simulink model "Modello_Irb1300"  (R2024a)
settings: Solver=VariableStepAuto  StartTime=0.0  StopTime=37  RelTol=1e-3
undefined symbols (not defined in the file or in its folder): DiscIntNeverNeededParam
libraries: vrlib x3, simulink x1
(part 1 of 2)
settings Model: Creator=giaki  LastModifiedBy=giaki

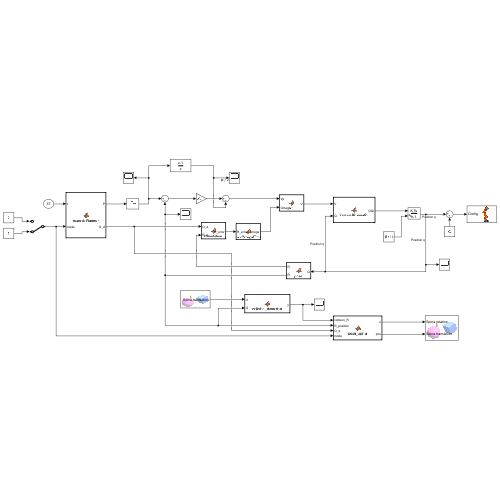
[thumbnail: Simulink's stored preview of the top-level diagram]
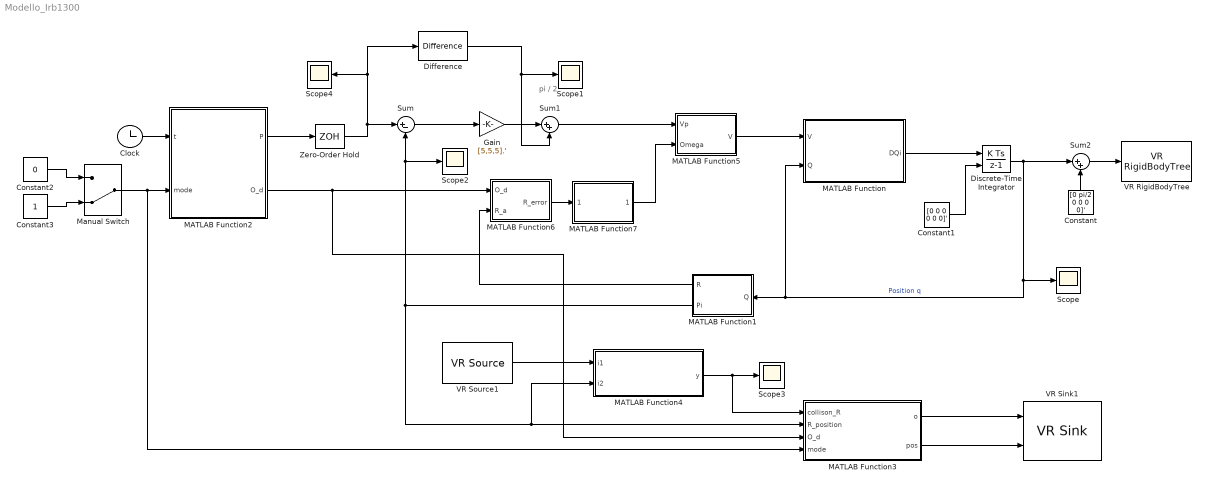
== system Modello_Irb1300 ==
  note: pi / 2
  Clock : Clock
  Constant : Constant  Value=[0 pi/2 0 0 0 0]'
  Constant1 : Constant  Value=[0 0 0 0 0 0]'
  Constant2 : Constant  Value=0
  Constant3 : Constant
  Difference : simulink/Discrete/Difference  ICPrevInput=[0.66, 0, 1.015].'  OutMin=[]  OutMax=[]  OutDataType=fixdt(1, 16)  OutScaling=2^-10  DoSatur=off
  Discrete-Time Integrator : DiscreteIntegrator  InitialConditionSource=external  SampleTime=-1  OutMin=[2]  ICPrevOutput=DiscIntNeverNeededParam  ICPrevScaledInput=DiscIntNeverNeededParam
  Gain : Gain  Gain=[5,5,5].'
  MATLAB Function : MATLAB Function  TreatAsAtomicUnit=on
  MATLAB Function1 : MATLAB Function  TreatAsAtomicUnit=on
  MATLAB Function2 : MATLAB Function  TreatAsAtomicUnit=on
  MATLAB Function3 : MATLAB Function  TreatAsAtomicUnit=on
  MATLAB Function4 : MATLAB Function  TreatAsAtomicUnit=on
  MATLAB Function5 : MATLAB Function  TreatAsAtomicUnit=on
  MATLAB Function6 : MATLAB Function  TreatAsAtomicUnit=on
  MATLAB Function7 : MATLAB Function  TreatAsAtomicUnit=on
  Manual Switch : ManualSwitch  CurrentSetting=0
  Scope{,1..4} (5 alike) : Scope
  Sum : Sum  Inputs=|+-
  Sum1 : Sum  Inputs=|++
  Sum2 : Sum  Inputs=|++
  VR RigidBodyTree : vrlib/VR RigidBodyTree  VrmlFile=robot_scene_2.x3d  RBT=Irb1300  useRBT=on  Ts=0.1  ForceViewerOpen=on
  VR Sink1 : vrlib/VR Sink  InstantiateOnLoad=on  SampleTime=0.1  ViewEnable=on  RemoteChange=off  RemoteView=off  FieldsWritten=Spina.rotation.4.1.1.double#Spina.translation.3.1.1.double  WorldFileName=robot_scene_2.x3d  WorldDescription=Simple Robot Scene  AutoView=off  VideoDimensions=[]  AllowVariableSize=off
  VR Source1 : vrlib/VR Source  InstantiateOnLoad=on  SampleTime=0.1  ViewEnable=on  RemoteChange=off  RemoteView=off  FieldsRead=Spina.translation.1.3.1.double  WorldFileName=robot_scene_2.x3d  WorldDescription=Simple Robot Scene  AutoView=off  VideoDimensions=[]  AllowVariableSize=off
  Zero-Order Hold : ZeroOrderHold  SampleTime=0.05
  wires:
  Discrete-Time Integrator/1 -> Sum2/1, Scope/1, MATLAB Function/2(Q), MATLAB Function1/1(Q)  "Position q"
  Constant/1 -> Sum2/2
  Constant1/1 -> Discrete-Time Integrator/2
  Sum2/1 -> VR RigidBodyTree/1
  Difference/1 -> Sum1/2, Scope1/1
  Clock/1 -> MATLAB Function2/1(t)
  MATLAB Function/1(DQi) -> Discrete-Time Integrator/1
  Gain/1 -> Sum1/1
  MATLAB Function4/1(y) -> MATLAB Function3/1(collison_R), Scope3/1
  VR Source1/1 -> MATLAB Function4/1(i1)
  MATLAB Function2/1(P) -> Zero-Order Hold/1
  MATLAB Function3/2(pos) -> VR Sink1/2
  Zero-Order Hold/1 -> Scope4/1, Difference/1, Sum/1
  Sum/1 -> Gain/1
  MATLAB Function1/1(R) -> MATLAB Function6/2(R_a)
  Sum1/1 -> MATLAB Function5/1(Vp)
  MATLAB Function5/1(V) -> MATLAB Function/1(V)
  MATLAB Function6/1(R_error) -> MATLAB Function7/1(R_error)
  MATLAB Function7/1(omega) -> MATLAB Function5/2(Omega)
  MATLAB Function1/2(Pi) -> Sum/2, Scope2/1, MATLAB Function4/2(i2), MATLAB Function3/2(R_position)
  MATLAB Function2/2(O_d) -> MATLAB Function3/3(O_d), MATLAB Function6/1(O_d)
  MATLAB Function3/1(o) -> VR Sink1/1
  Manual Switch/1 -> MATLAB Function3/4(mode), MATLAB Function2/2(mode)
  Constant2/1 -> Manual Switch/1
  Constant3/1 -> Manual Switch/2

== matlab function Modello_Irb1300/MATLAB Function1 ==
  data: R output; Q input; Pi output


function [R,Pi] = posa(Q)

th1 = Q(1);
th2 = Q(2);
th3 = Q(3);
th4 = Q(4);
th5 = Q(5);
th6 = Q(6);

% Matrice di trasformazione 4x4 calcolata nella posizione Q
T = [
    [sin(th6)*(cos(th4)*sin(th1) + sin(th4)*(cos(th1)*sin(th3)*sin(th2 + pi/2) - cos(th1)*cos(th3)*cos(th2 + pi/2))) + cos(th6)*(cos(th5)*(sin(th1)*sin(th4) - cos(th4)*(cos(th1)*sin(th3)*sin(th2 + pi/2) - cos(th1)*cos(th3)*cos(th2 + pi/2))) - sin(th5)*(cos(th1)*cos(th3)*sin(th2 + pi/2) + cos(th1)*cos(th2 + pi/2)*sin(th3))), cos(th6)*(cos(th4)*sin(th1) + sin(th4)*(cos(th1)*sin(th3)*sin(th2 + pi/2) - cos(th1)*cos(th3)*cos(th2 + pi/2))) - sin(th6)*(cos(th5)*(sin(th1)*sin(th4) - cos(th4)*(cos(th1)*sin(th3)*sin(th2 + pi/2) - cos(th1)*cos(th3)*cos(th2 + pi/2))) - sin(th5)*(cos(th1)*cos(th3)*sin(th2 + pi/2) + cos(th1)*cos(th2 + pi/2)*sin(th3))), sin(th5)*(sin(th1)*sin(th4) - cos(th4)*(cos(th1)*sin(th3)*sin(th2 + pi/2) - cos(th1)*cos(th3)*cos(th2 + pi/2))) + cos(th5)*(cos(th1)*cos(th3)*sin(th2 + pi/2) + cos(th1)*cos(th2 + pi/2)*sin(th3)), cos(th1)/20 + (17*cos(th1)*cos(th2 + pi/2))/40 + (9*sin(th5)*(sin(th1)*sin(th4) - cos(th4)*(cos(th1)*sin(th3)*sin(th2 + pi/2) - cos(th1)*cos(th3)*cos(th2 + pi/2))))/50 + (9*cos(th5)*(cos(th1)*cos(th3)*sin(th2 + pi/2) + cos(th1)*cos(th2 + pi/2)*sin(th3)))/50 + (17*cos(th1)*cos(th3)*sin(th2 + pi/2))/40 + (17*cos(th1)*cos(th2 + pi/2)*sin(th3))/40 - (cos(th1)*sin(th3)*sin(th2 + pi/2))/25 + (cos(th1)*cos(th3)*cos(th2 + pi/2))/25]
    [-sin(th6)*(cos(th1)*cos(th4) + sin(th4)*(cos(th3)*cos(th2 + pi/2)*sin(th1) - sin(th1)*sin(th3)*sin(th2 + pi/2))) - cos(th6)*(cos(th5)*(cos(th1)*sin(th4) - cos(th4)*(cos(th3)*cos(th2 + pi/2)*sin(th1) - sin(th1)*sin(th3)*sin(th2 + pi/2))) + sin(th5)*(cos(th3)*sin(th1)*sin(th2 + pi/2) + cos(th2 + pi/2)*sin(th1)*sin(th3))), sin(th6)*(cos(th5)*(cos(th1)*sin(th4) - cos(th4)*(cos(th3)*cos(th2 + pi/2)*sin(th1) - sin(th1)*sin(th3)*sin(th2 + pi/2))) + sin(th5)*(cos(th3)*sin(th1)*sin(th2 + pi/2) + cos(th2 + pi/2)*sin(th1)*sin(th3))) - cos(th6)*(cos(th1)*cos(th4) + sin(th4)*(cos(th3)*cos(th2 + pi/2)*sin(th1) - sin(th1)*sin(th3)*sin(th2 + pi/2))), cos(th5)*(cos(th3)*sin(th1)*sin(th2 + pi/2) + cos(th2 + pi/2)*sin(th1)*sin(th3)) - sin(th5)*(cos(th1)*sin(th4) - cos(th4)*(cos(th3)*cos(th2 + pi/2)*sin(th1) - sin(th1)*sin(th3)*sin(th2 + pi/2))), sin(th1)/20 + (17*cos(th2 + pi/2)*sin(th1))/40 - (9*sin(th5)*(cos(th1)*sin(th4) - cos(th4)*(cos(th3)*cos(th2 + pi/2)*sin(th1) - sin(th1)*sin(th3)*sin(th2 + pi/2))))/50 + (9*cos(th5)*(cos(th3)*sin(th1)*sin(th2 + pi/2) + cos(th2 + pi/2)*sin(th1)*sin(th3)))/50 + (cos(th3)*cos(th2 + pi/2)*sin(th1))/25 + (17*cos(th3)*sin(th1)*sin(th2 + pi/2))/40 + (17*cos(th2 + pi/2)*sin(th1)*sin(th3))/40 - (sin(th1)*sin(th3)*sin(th2 + pi/2))/25]
    [cos(th6)*(sin(th5)*(cos(th3)*cos(th2 + pi/2) - sin(th3)*sin(th2 + pi/2)) + cos(th4)*cos(th5)*(cos(th3)*sin(th2 + pi/2) + cos(th2 + pi/2)*sin(th3))) - sin(th4)*sin(th6)*(cos(th3)*sin(th2 + pi/2) + cos(th2 + pi/2)*sin(th3)), -sin(th6)*(sin(th5)*(cos(th3)*cos(th2 + pi/2) - sin(th3)*sin(th2 + pi/2)) + cos(th4)*cos(th5)*(cos(th3)*sin(th2 + pi/2) + cos(th2 + pi/2)*sin(th3))) - cos(th6)*sin(th4)*(cos(th3)*sin(th2 + pi/2) + cos(th2 + pi/2)*sin(th3)), cos(th4)*sin(th5)*(cos(th3)*sin(th2 + pi/2) + cos(th2 + pi/2)*sin(th3)) - cos(th5)*(cos(th3)*cos(th2 + pi/2) - sin(th3)*sin(th2 + pi/2)), (17*sin(th2 + pi/2))/40 - (17*cos(th3)*cos(th2 + pi/2))/40 + (cos(th3)*sin(th2 + pi/2))/25 + (cos(th2 + pi/2)*sin(th3))/25 + (17*sin(th3)*sin(th2 + pi/2))/40 - (9*cos(th5)*(cos(th3)*cos(th2 + pi/2) - sin(th3)*sin(th2 + pi/2)))/50 + (9*cos(th4)*sin(th5)*(cos(th3)*sin(th2 + pi/2) + cos(th2 + pi/2)*sin(th3)))/50 + 68/125]
    [0, 0, 0, 1]
];

% Estrai la posizione (3x1)
Pi_position = T(1:3, 4);

% Estrai la matrice di rotazione (3x3)
R = T(1:3, 1:3);

% % Calcola Roll, Pitch, Yaw dalla matrice di rotazione
% roll = atan2(R(3,2), R(3,3));   % Roll (x)
% pitch = atan2(-R(3,1), sqrt(R(3,2)^2 + R(3,3)^2));  % Pitch (y)
% yaw = atan2(R(2,1), R(1,1));    % Yaw (z)
% 
% % Mantieni roll, pitch, yaw nel range [-π, π]
% roll = wrapToPi(roll);
% pitch = wrapToPi(pitch);
% yaw = wrapToPi(yaw);

% Restituisci la posizione e l'orientamento come un vettore 6x1
%Pi = [Pi_position; roll; pitch; yaw];
%Pi = [Pi_position; R(:,3)];
Pi = [Pi_position];
% end













% function Pi = posa(Q)
% 
% th1 = Q(1);
% th2 = Q(2);
% th3 = Q(3);
% th4 = Q(4);
% th5 = Q(5);
% th6 = Q(6);
% 
% % matrix 4x4 evaluated in the position Q
% % matriceUtilizzata T06 calcolata con la terna di riferimento posizionata
% % sul punto di aggancio della pinza 
% T = [
% [  sin(th6)*(cos(th4)*sin(th1) + sin(th4)*(cos(th1)*sin(th3)*sin(th2 + pi/2) - cos(th1)*cos(th3)*cos(th2 + pi/2))) + cos(th6)*(cos(th5)*(sin(th1)*sin(th4) - cos(th4)*(cos(th1)*sin(th3)*sin(th2 + pi/2) - cos(th1)*cos(th3)*cos(th2 + pi/2))) - sin(th5)*(cos(th1)*cos(th3)*sin(th2 + pi/2) + cos(th1)*cos(th2 + pi/2)*sin(th3))), cos(th6)*(cos(th4)*sin(th1) + sin(th4)*(cos(th1)*sin(th3)*sin(th2 + pi/2) - cos(th1)*cos(th3)*cos(th2 + pi/2))) - sin(th6)*(cos(th5)*(sin(th1)*sin(th4) - cos(th4)*(cos(th1)*sin(th3)*sin(th2 + pi/2) - cos(th1)*cos(th3)*cos(th2 + pi/2))) - sin(th5)*(cos(th1)*cos(th3)*sin(th2 + pi/2) + cos(th1)*cos(th2 + pi/2)*sin(th3))), sin(th5)*(sin(th1)*sin(th4) - cos(th4)*(cos(th1)*sin(th3)*sin(th2 + pi/2) - cos(th1)*cos(th3)*cos(th2 + pi/2))) + cos(th5)*(cos(th1)*cos(th3)*sin(th2 + pi/2) + cos(th1)*cos(th2 + pi/2)*sin(th3)), cos(th1)/20 + (17*cos(th1)*cos(th2 + pi/2))/40 + (9*sin(th5)*(sin(th1)*sin(th4) - cos(th4)*(cos(th1)*sin(th3)*sin(th2 + pi/2) - cos(th1)*cos(th3)*cos(th2 + pi/2))))/50 + (9*cos(th5)*(cos(th1)*cos(th3)*sin(th2 + pi/2) + cos(th1)*cos(th2 + pi/2)*sin(th3)))/50 + (17*cos(th1)*cos(th3)*sin(th2 + pi/2))/40 + (17*cos(th1)*cos(th2 + pi/2)*sin(th3))/40 - (cos(th1)*sin(th3)*sin(th2 + pi/2))/25 + (cos(th1)*cos(th3)*cos(th2 + pi/2))/25]
% [- sin(th6)*(cos(th1)*cos(th4) + sin(th4)*(cos(th3)*cos(th2 + pi/2)*sin(th1) - sin(th1)*sin(th3)*sin(th2 + pi/2))) - cos(th6)*(cos(th5)*(cos(th1)*sin(th4) - cos(th4)*(cos(th3)*cos(th2 + pi/2)*sin(th1) - sin(th1)*sin(th3)*sin(th2 + pi/2))) + sin(th5)*(cos(th3)*sin(th1)*sin(th2 + pi/2) + cos(th2 + pi/2)*sin(th1)*sin(th3))), sin(th6)*(cos(th5)*(cos(th1)*sin(th4) - cos(th4)*(cos(th3)*cos(th2 + pi/2)*sin(th1) - sin(th1)*sin(th3)*sin(th2 + pi/2))) + sin(th5)*(cos(th3)*sin(th1)*sin(th2 + pi/2) + cos(th2 + pi/2)*sin(th1)*sin(th3))) - cos(th6)*(cos(th1)*cos(th4) + sin(th4)*(cos(th3)*cos(th2 + pi/2)*sin(th1) - sin(th1)*sin(th3)*sin(th2 + pi/2))), cos(th5)*(cos(th3)*sin(th1)*sin(th2 + pi/2) + cos(th2 + pi/2)*sin(th1)*sin(th3)) - sin(th5)*(cos(th1)*sin(th4) - cos(th4)*(cos(th3)*cos(th2 + pi/2)*sin(th1) - sin(th1)*sin(th3)*sin(th2 + pi/2))), sin(th1)/20 + (17*cos(th2 + pi/2)*sin(th1))/40 - (9*sin(th5)*(cos(th1)*sin(th4) - cos(th4)*(cos(th3)*cos(th2 + pi/2)*sin(th1) - sin(th1)*sin(th3)*sin(th2 + pi/2))))/50 + (9*cos(th5)*(cos(th3)*sin(th1)*sin(th2 + pi/2) + cos(th2 + pi/2)*sin(th1)*sin(th3)))/50 + (cos(th3)*cos(th2 + pi/2)*sin(th1))/25 + (17*cos(th3)*sin(th1)*sin(th2 + pi/2))/40 + (17*cos(th2 + pi/2)*sin(th1)*sin(th3))/40 - (sin(th1)*sin(th3)*sin(th2 + pi/2))/25]
% [                                                                                                    cos(th6)*(sin(th5)*(cos(th3)*cos(th2 + pi/2) - sin(th3)*sin(th2 + pi/2)) + cos(th4)*cos(th5)*(cos(th3)*sin(th2 + pi/2) + cos(th2 + pi/2)*sin(th3))) - sin(th4)*sin(th6)*(cos(th3)*sin(th2 + pi/2) + cos(th2 + pi/2)*sin(th3)),                                                                                                 - sin(th6)*(sin(th5)*(cos(th3)*cos(th2 + pi/2) - sin(th3)*sin(th2 + pi/2)) + cos(th4)*cos(th5)*(cos(th3)*sin(th2 + pi/2) + cos(th2 + pi/2)*sin(th3))) - cos(th6)*sin(th4)*(cos(th3)*sin(th2 + pi/2) + cos(th2 + pi/2)*sin(th3)),                                                           cos(th4)*sin(th5)*(cos(th3)*sin(th2 + pi/2) + cos(th2 + pi/2)*sin(th3)) - cos(th5)*(cos(th3)*cos(th2 + pi/2) - sin(th3)*sin(th2 + pi/2)),                                                                                                             (17*sin(th2 + pi/2))/40 - (17*cos(th3)*cos(th2 + pi/2))/40 + (cos(th3)*sin(th2 + pi/2))/25 + (cos(th2 + pi/2)*sin(th3))/25 + (17*sin(th3)*sin(th2 + pi/2))/40 - (9*cos(th5)*(cos(th3)*cos(th2 + pi/2) - sin(th3)*sin(th2 + pi/2)))/50 + (9*cos(th4)*sin(th5)*(cos(th3)*sin(th2 + pi/2) + cos(th2 + pi/2)*sin(th3)))/50 + 68/125]
% [                                                                                                                                                                                                                                                                                                                                0,                                                                                                                                                                                                                                                                                                                               0,                                                                                                                                                                                                  0,                                                                                                                                                                                                                                                                                                                                                                                                                                           1]
%  ];
% 
% % T = [
% % [  sin(th6)*(cos(th4)*sin(th1) + sin(th4)*(cos(th1)*sin(th3)*sin(th2 + pi/2) - cos(th1)*cos(th3)*cos(th2 + pi/2))) + cos(th6)*(cos(th5)*(sin(th1)*sin(th4) - cos(th4)*(cos(th1)*sin(th3)*sin(th2 + pi/2) - cos(th1)*cos(th3)*cos(th2 + pi/2))) - sin(th5)*(cos(th1)*cos(th3)*sin(th2 + pi/2) + cos(th1)*cos(th2 + pi/2)*sin(th3))), cos(th6)*(cos(th4)*sin(th1) + sin(th4)*(cos(th1)*sin(th3)*sin(th2 + pi/2) - cos(th1)*cos(th3)*cos(th2 + pi/2))) - sin(th6)*(cos(th5)*(sin(th1)*sin(th4) - cos(th4)*(cos(th1)*sin(th3)*sin(th2 + pi/2) - cos(th1)*cos(th3)*cos(th2 + pi/2))) - sin(th5)*(cos(th1)*cos(th3)*sin(th2 + pi/2) + cos(th1)*cos(th2 + pi/2)*sin(th3))), sin(th5)*(sin(th1)*sin(th4) - cos(th4)*(cos(th1)*sin(th3)*sin(th2 + pi/2) - cos(th1)*cos(th3)*cos(th2 + pi/2))) + cos(th5)*(cos(th1)*cos(th3)*sin(th2 + pi/2) + cos(th1)*cos(th2 + pi/2)*sin(th3)), cos(th1)/20 + (17*cos(th1)*cos(th2 + pi/2))/40 + (9*sin(th5)*(sin(th1)*sin(th4) - cos(th4)*(cos(th1)*sin(th3)*sin(th2 + pi/2) - cos(th1)*cos(th3)*cos(th2 + pi/2))))/100 + (9*cos(th5)*(cos(th1)*cos(th3)*sin(th2 + pi/2) + cos(th1)*cos(th2 + pi/2)*sin(th3)))/100 + (17*cos(th1)*cos(th3)*sin(th2 + pi/2))/40 + (17*cos(th1)*cos(th2 + pi/2)*sin(th3))/40 - (cos(th1)*sin(th3)*sin(th2 + pi/2))/25 + (cos(th1)*cos(th3)*cos(th2 + pi/2))/25]
% % [- sin(th6)*(cos(th1)*cos(th4) + sin(th4)*(cos(th3)*cos(th2 + pi/2)*sin(th1) - sin(th1)*sin(th3)*sin(th2 + pi/2))) - cos(th6)*(cos(th5)*(cos(th1)*sin(th4) - cos(th4)*(cos(th3)*cos(th2 + pi/2)*sin(th1) - sin(th1)*sin(th3)*sin(th2 + pi/2))) + sin(th5)*(cos(th3)*sin(th1)*sin(th2 + pi/2) + cos(th2 + pi/2)*sin(th1)*sin(th3))), sin(th6)*(cos(th5)*(cos(th1)*sin(th4) - cos(th4)*(cos(th3)*cos(th2 + pi/2)*sin(th1) - sin(th1)*sin(th3)*sin(th2 + pi/2))) + sin(th5)*(cos(th3)*sin(th1)*sin(th2 + pi/2) + cos(th2 + pi/2)*sin(th1)*sin(th3))) - cos(th6)*(cos(th1)*cos(th4) + sin(th4)*(cos(th3)*cos(th2 + pi/2)*sin(th1) - sin(th1)*sin(th3)*sin(th2 + pi/2))), cos(th5)*(cos(th3)*sin(th1)*sin(th2 + pi/2) + cos(th2 + pi/2)*sin(th1)*sin(th3)) - sin(th5)*(cos(th1)*sin(th4) - cos(th4)*(cos(th3)*cos(th2 + pi/2)*sin(th1) - sin(th1)*sin(th3)*sin(th2 + pi/2))), sin(th1)/20 + (17*cos(th2 + pi/2)*sin(th1))/40 - (9*sin(th5)*(cos(th1)*sin(th4) - cos(th4)*(cos(th3)*cos(th2 + pi/2)*sin(th1) - sin(th1)*sin(th3)*sin(th2 + pi/2))))/100 + (9*cos(th5)*(cos(th3)*sin(th1)*sin(th2 + pi/2) + cos(th2 + pi/2)*sin(th1)*sin(th3)))/100 + (cos(th3)*cos(th2 + pi/2)*sin(th1))/25 + (17*cos(th3)*sin(th1)*sin(th2 + pi/2))/40 + (17*cos(th2 + pi/2)*sin(th1)*sin(th3))/40 - (sin(th1)*sin(th3)*sin(th2 + pi/2))/25]
% % [                                                                                                    cos(th6)*(sin(th5)*(cos(th3)*cos(th2 + pi/2) - sin(th3)*sin(th2 + pi/2)) + cos(th4)*cos(th5)*(cos(th3)*sin(th2 + pi/2) + cos(th2 + pi/2)*sin(th3))) - sin(th4)*sin(th6)*(cos(th3)*sin(th2 + pi/2) + cos(th2 + pi/2)*sin(th3)),                                                                                                 - sin(th6)*(sin(th5)*(cos(th3)*cos(th2 + pi/2) - sin(th3)*sin(th2 + pi/2)) + cos(th4)*cos(th5)*(cos(th3)*sin(th2 + pi/2) + cos(th2 + pi/2)*sin(th3))) - cos(th6)*sin(th4)*(cos(th3)*sin(th2 + pi/2) + cos(th2 + pi/2)*sin(th3)),                                                           cos(th4)*sin(th5)*(cos(th3)*sin(th2 + pi/2) + cos(th2 + pi/2)*sin(th3)) - cos(th5)*(cos(th3)*cos(th2 + pi/2) - sin(th3)*sin(th2 + pi/2)),                                                                                                             (17*sin(th2 + pi/2))/40 - (17*cos(th3)*cos(th2 + pi/2))/40 + (cos(th3)*sin(th2 + pi/2))/25 + (cos(th2 + pi/2)*sin(th3))/25 + (17*sin(th3)*sin(th2 + pi/2))/40 - (9*cos(th5)*(cos(th3)*cos(th2 + pi/2) - sin(th3)*sin(th2 + pi/2)))/100 + (9*cos(th4)*sin(th5)*(cos(th3)*sin(th2 + pi/2) + cos(th2 + pi/2)*sin(th3)))/100 + 68/125]
% % [                                                                                                                                                                                                                                                                                                                                0,                                                                                                                                                                                                                                                                                                                               0,                                                                                                                                                                                                  0,                                                                                                                                                                                                                                                                                                                                                                                                                                             1]
% % ];
% 
% 
% % Estrai la posizione (3x1)
% Pi_position = T(1:3, 4);
% 
% % Estrai la matrice di rotazione (3x3)
% R = T(1:3, 1:3);
% 
% % % Calcola Roll, Pitch, Yaw dalla matrice di rotazione
% roll = atan2(R(3,2), R(3,3));   % Roll (x)
% pitch = atan2(-R(3,1), sqrt(R(3,2)^2 + R(3,3)^2));  % Pitch (y)
% yaw = atan2(R(2,1), R(1,1));    % Yaw (z)
% 
% % Restituisci la posizione e l'orientamento come un vettore 6x1%
% Pi = [Pi_position; roll; pitch; yaw];  % iniziale 
% %Pi = [Pi_position; yaw; pitch; roll];  % Test
% %Pi = [Pi_position; pitch; yaw; roll];
% %Pi = [Pi_position];
% end

== matlab function Modello_Irb1300/MATLAB Function ==
  data: V input; DQi output; Q input
function DQi = inverseKinematic(V,Q)

th1 = Q(1);
th2 = Q(2);
th3 = Q(3);
th4 = Q(4);
th5 = Q(5);
th6 = Q(6);



% cosiderando sia le traslazioni che le orientazioni viene utilizzato il seguente J che si riferisce al jacobiano completo J = Jp + Jo 
J = [
[(9*sin(th5)*(cos(th1)*sin(th4) - cos(th4)*(cos(th3)*cos(th2 + pi/2)*sin(th1) - sin(th1)*sin(th3)*sin(th2 + pi/2))))/50 - (17*cos(th2 + pi/2)*sin(th1))/40 - sin(th1)/20 - (9*cos(th5)*(cos(th3)*sin(th1)*sin(th2 + pi/2) + cos(th2 + pi/2)*sin(th1)*sin(th3)))/50 - (cos(th3)*cos(th2 + pi/2)*sin(th1))/25 - (17*cos(th3)*sin(th1)*sin(th2 + pi/2))/40 - (17*cos(th2 + pi/2)*sin(th1)*sin(th3))/40 + (sin(th1)*sin(th3)*sin(th2 + pi/2))/25, (17*cos(th1)*cos(th3)*cos(th2 + pi/2))/40 - (9*cos(th5)*(cos(th1)*sin(th3)*sin(th2 + pi/2) - cos(th1)*cos(th3)*cos(th2 + pi/2)))/50 - (cos(th1)*cos(th3)*sin(th2 + pi/2))/25 - (cos(th1)*cos(th2 + pi/2)*sin(th3))/25 - (17*cos(th1)*sin(th3)*sin(th2 + pi/2))/40 - (9*cos(th4)*sin(th5)*(cos(th1)*cos(th3)*sin(th2 + pi/2) + cos(th1)*cos(th2 + pi/2)*sin(th3)))/50 - (17*cos(th1)*sin(th2 + pi/2))/40, (17*cos(th1)*cos(th3)*cos(th2 + pi/2))/40 - (cos(th1)*cos(th3)*sin(th2 + pi/2))/25 - (cos(th1)*cos(th2 + pi/2)*sin(th3))/25 - (17*cos(th1)*sin(th3)*sin(th2 + pi/2))/40 - (9*cos(th4)*sin(th5)*(cos(th1)*cos(th3)*sin(th2 + pi/2) + cos(th1)*cos(th2 + pi/2)*sin(th3)))/50 - (9*cos(th5)*(cos(th1)*sin(th3)*sin(th2 + pi/2) - cos(th1)*cos(th3)*cos(th2 + pi/2)))/50,  (9*sin(th5)*(cos(th4)*sin(th1) + sin(th4)*(cos(th1)*sin(th3)*sin(th2 + pi/2) - cos(th1)*cos(th3)*cos(th2 + pi/2))))/50,   (9*cos(th5)*(sin(th1)*sin(th4) - cos(th4)*(cos(th1)*sin(th3)*sin(th2 + pi/2) - cos(th1)*cos(th3)*cos(th2 + pi/2))))/50 - (9*sin(th5)*(cos(th1)*cos(th3)*sin(th2 + pi/2) + cos(th1)*cos(th2 + pi/2)*sin(th3)))/50,                                                                                                                                                                                                  0]
[cos(th1)/20 + (17*cos(th1)*cos(th2 + pi/2))/40 + (9*sin(th5)*(sin(th1)*sin(th4) - cos(th4)*(cos(th1)*sin(th3)*sin(th2 + pi/2) - cos(th1)*cos(th3)*cos(th2 + pi/2))))/50 + (9*cos(th5)*(cos(th1)*cos(th3)*sin(th2 + pi/2) + cos(th1)*cos(th2 + pi/2)*sin(th3)))/50 + (17*cos(th1)*cos(th3)*sin(th2 + pi/2))/40 + (17*cos(th1)*cos(th2 + pi/2)*sin(th3))/40 - (cos(th1)*sin(th3)*sin(th2 + pi/2))/25 + (cos(th1)*cos(th3)*cos(th2 + pi/2))/25, (9*cos(th5)*(cos(th3)*cos(th2 + pi/2)*sin(th1) - sin(th1)*sin(th3)*sin(th2 + pi/2)))/50 - (17*sin(th1)*sin(th2 + pi/2))/40 + (17*cos(th3)*cos(th2 + pi/2)*sin(th1))/40 - (cos(th3)*sin(th1)*sin(th2 + pi/2))/25 - (cos(th2 + pi/2)*sin(th1)*sin(th3))/25 - (17*sin(th1)*sin(th3)*sin(th2 + pi/2))/40 - (9*cos(th4)*sin(th5)*(cos(th3)*sin(th1)*sin(th2 + pi/2) + cos(th2 + pi/2)*sin(th1)*sin(th3)))/50, (9*cos(th5)*(cos(th3)*cos(th2 + pi/2)*sin(th1) - sin(th1)*sin(th3)*sin(th2 + pi/2)))/50 + (17*cos(th3)*cos(th2 + pi/2)*sin(th1))/40 - (cos(th3)*sin(th1)*sin(th2 + pi/2))/25 - (cos(th2 + pi/2)*sin(th1)*sin(th3))/25 - (17*sin(th1)*sin(th3)*sin(th2 + pi/2))/40 - (9*cos(th4)*sin(th5)*(cos(th3)*sin(th1)*sin(th2 + pi/2) + cos(th2 + pi/2)*sin(th1)*sin(th3)))/50, -(9*sin(th5)*(cos(th1)*cos(th4) + sin(th4)*(cos(th3)*cos(th2 + pi/2)*sin(th1) - sin(th1)*sin(th3)*sin(th2 + pi/2))))/50, - (9*cos(th5)*(cos(th1)*sin(th4) - cos(th4)*(cos(th3)*cos(th2 + pi/2)*sin(th1) - sin(th1)*sin(th3)*sin(th2 + pi/2))))/50 - (9*sin(th5)*(cos(th3)*sin(th1)*sin(th2 + pi/2) + cos(th2 + pi/2)*sin(th1)*sin(th3)))/50,                                                                                                                                                                                                  0]
[                                                                                                                                                                                                                                                                                                                                                                                                                                          0,                                                                                  (17*cos(th2 + pi/2))/40 + (cos(th3)*cos(th2 + pi/2))/25 + (17*cos(th3)*sin(th2 + pi/2))/40 + (17*cos(th2 + pi/2)*sin(th3))/40 - (sin(th3)*sin(th2 + pi/2))/25 + (9*cos(th5)*(cos(th3)*sin(th2 + pi/2) + cos(th2 + pi/2)*sin(th3)))/50 + (9*cos(th4)*sin(th5)*(cos(th3)*cos(th2 + pi/2) - sin(th3)*sin(th2 + pi/2)))/50,                                                                         (cos(th3)*cos(th2 + pi/2))/25 + (17*cos(th3)*sin(th2 + pi/2))/40 + (17*cos(th2 + pi/2)*sin(th3))/40 - (sin(th3)*sin(th2 + pi/2))/25 + (9*cos(th5)*(cos(th3)*sin(th2 + pi/2) + cos(th2 + pi/2)*sin(th3)))/50 + (9*cos(th4)*sin(th5)*(cos(th3)*cos(th2 + pi/2) - sin(th3)*sin(th2 + pi/2)))/50,                                         -(9*sin(th4)*sin(th5)*(cos(th3)*sin(th2 + pi/2) + cos(th2 + pi/2)*sin(th3)))/50,                                                             (9*sin(th5)*(cos(th3)*cos(th2 + pi/2) - sin(th3)*sin(th2 + pi/2)))/50 + (9*cos(th4)*cos(th5)*(cos(th3)*sin(th2 + pi/2) + cos(th2 + pi/2)*sin(th3)))/50,                                                                                                                                                                                                  0]
[                                                                                                                                                                                                                                                                                                                                                                                                                                          0,                                                                                                                                                                                                                                                                                                                                                                                                sin(th1),                                                                                                                                                                                                                                                                                                                                                             sin(th1),                                                   cos(th1)*cos(th3)*sin(th2 + pi/2) + cos(th1)*cos(th2 + pi/2)*sin(th3),                                                                                                               cos(th4)*sin(th1) + sin(th4)*(cos(th1)*sin(th3)*sin(th2 + pi/2) - cos(th1)*cos(th3)*cos(th2 + pi/2)), sin(th5)*(sin(th1)*sin(th4) - cos(th4)*(cos(th1)*sin(th3)*sin(th2 + pi/2) - cos(th1)*cos(th3)*cos(th2 + pi/2))) + cos(th5)*(cos(th1)*cos(th3)*sin(th2 + pi/2) + cos(th1)*cos(th2 + pi/2)*sin(th3))]
[                                                                                                                                                                                                                                                                                                                                                                                                                                          0,                                                                                                                                                                                                                                                                                                                                                                                               -cos(th1),                                                                                                                                                                                                                                                                                                                                                            -cos(th1),                                                   cos(th3)*sin(th1)*sin(th2 + pi/2) + cos(th2 + pi/2)*sin(th1)*sin(th3),                                                                                                             - cos(th1)*cos(th4) - sin(th4)*(cos(th3)*cos(th2 + pi/2)*sin(th1) - sin(th1)*sin(th3)*sin(th2 + pi/2)), cos(th5)*(cos(th3)*sin(th1)*sin(th2 + pi/2) + cos(th2 + pi/2)*sin(th1)*sin(th3)) - sin(th5)*(cos(th1)*sin(th4) - cos(th4)*(cos(th3)*cos(th2 + pi/2)*sin(th1) - sin(th1)*sin(th3)*sin(th2 + pi/2)))]
[                                                                                                                                                                                                                                                                                                                                                                                                                                          1,                                                                                                                                                                                                                                                                                                                                                                                                       0,                                                                                                                                                                                                                                                                                                                                                                    0,                                                                     sin(th3)*sin(th2 + pi/2) - cos(th3)*cos(th2 + pi/2),                                                                                                                                                    -sin(th4)*(cos(th3)*sin(th2 + pi/2) + cos(th2 + pi/2)*sin(th3)),                                                           cos(th4)*sin(th5)*(cos(th3)*sin(th2 + pi/2) + cos(th2 + pi/2)*sin(th3)) - cos(th5)*(cos(th3)*cos(th2 + pi/2) - sin(th3)*sin(th2 + pi/2))]
];



DQi = pinv(J)*V; % Matlab function for thr pseudo-inverse Matrix
pause (0.01);

end






% Jacobian evaluated every time in the position Q

% calcolato con la terna posizionata sul punto di aggancio della pinza 
% Considerando solo le traslazioni viene utilizzato Jp scriviamo J ma il jacobiano seguente è in verità il jacobiano di
% poszione Jp 

% J = [
% 
% [(9*sin(th5)*(cos(th1)*sin(th4) - cos(th4)*(cos(th3)*cos(th2 + pi/2)*sin(th1) - sin(th1)*sin(th3)*sin(th2 + pi/2))))/50 - (17*cos(th2 + pi/2)*sin(th1))/40 - sin(th1)/20 - (9*cos(th5)*(cos(th3)*sin(th1)*sin(th2 + pi/2) + cos(th2 + pi/2)*sin(th1)*sin(th3)))/50 - (cos(th3)*cos(th2 + pi/2)*sin(th1))/25 - (17*cos(th3)*sin(th1)*sin(th2 + pi/2))/40 - (17*cos(th2 + pi/2)*sin(th1)*sin(th3))/40 + (sin(th1)*sin(th3)*sin(th2 + pi/2))/25, (17*cos(th1)*cos(th3)*cos(th2 + pi/2))/40 - (9*cos(th5)*(cos(th1)*sin(th3)*sin(th2 + pi/2) - cos(th1)*cos(th3)*cos(th2 + pi/2)))/50 - (cos(th1)*cos(th3)*sin(th2 + pi/2))/25 - (cos(th1)*cos(th2 + pi/2)*sin(th3))/25 - (17*cos(th1)*sin(th3)*sin(th2 + pi/2))/40 - (9*cos(th4)*sin(th5)*(cos(th1)*cos(th3)*sin(th2 + pi/2) + cos(th1)*cos(th2 + pi/2)*sin(th3)))/50 - (17*cos(th1)*sin(th2 + pi/2))/40, (17*cos(th1)*cos(th3)*cos(th2 + pi/2))/40 - (cos(th1)*cos(th3)*sin(th2 + pi/2))/25 - (cos(th1)*cos(th2 + pi/2)*sin(th3))/25 - (17*cos(th1)*sin(th3)*sin(th2 + pi/2))/40 - (9*cos(th4)*sin(th5)*(cos(th1)*cos(th3)*sin(th2 + pi/2) + cos(th1)*cos(th2 + pi/2)*sin(th3)))/50 - (9*cos(th5)*(cos(th1)*sin(th3)*sin(th2 + pi/2) - cos(th1)*cos(th3)*cos(th2 + pi/2)))/50,  (9*sin(th5)*(cos(th4)*sin(th1) + sin(th4)*(cos(th1)*sin(th3)*sin(th2 + pi/2) - cos(th1)*cos(th3)*cos(th2 + pi/2))))/50,   (9*cos(th5)*(sin(th1)*sin(th4) - cos(th4)*(cos(th1)*sin(th3)*sin(th2 + pi/2) - cos(th1)*cos(th3)*cos(th2 + pi/2))))/50 - (9*sin(th5)*(cos(th1)*cos(th3)*sin(th2 + pi/2) + cos(th1)*cos(th2 + pi/2)*sin(th3)))/50, 0]
% [cos(th1)/20 + (17*cos(th1)*cos(th2 + pi/2))/40 + (9*sin(th5)*(sin(th1)*sin(th4) - cos(th4)*(cos(th1)*sin(th3)*sin(th2 + pi/2) - cos(th1)*cos(th3)*cos(th2 + pi/2))))/50 + (9*cos(th5)*(cos(th1)*cos(th3)*sin(th2 + pi/2) + cos(th1)*cos(th2 + pi/2)*sin(th3)))/50 + (17*cos(th1)*cos(th3)*sin(th2 + pi/2))/40 + (17*cos(th1)*cos(th2 + pi/2)*sin(th3))/40 - (cos(th1)*sin(th3)*sin(th2 + pi/2))/25 + (cos(th1)*cos(th3)*cos(th2 + pi/2))/25, (9*cos(th5)*(cos(th3)*cos(th2 + pi/2)*sin(th1) - sin(th1)*sin(th3)*sin(th2 + pi/2)))/50 - (17*sin(th1)*sin(th2 + pi/2))/40 + (17*cos(th3)*cos(th2 + pi/2)*sin(th1))/40 - (cos(th3)*sin(th1)*sin(th2 + pi/2))/25 - (cos(th2 + pi/2)*sin(th1)*sin(th3))/25 - (17*sin(th1)*sin(th3)*sin(th2 + pi/2))/40 - (9*cos(th4)*sin(th5)*(cos(th3)*sin(th1)*sin(th2 + pi/2) + cos(th2 + pi/2)*sin(th1)*sin(th3)))/50, (9*cos(th5)*(cos(th3)*cos(th2 + pi/2)*sin(th1) - sin(th1)*sin(th3)*sin(th2 + pi/2)))/50 + (17*cos(th3)*cos(th2 + pi/2)*sin(th1))/40 - (cos(th3)*sin(th1)*sin(th2 + pi/2))/25 - (cos(th2 + pi/2)*sin(th1)*sin(th3))/25 - (17*sin(th1)*sin(th3)*sin(th2 + pi/2))/40 - (9*cos(th4)*sin(th5)*(cos(th3)*sin(th1)*sin(th2 + pi/2) + cos(th2 + pi/2)*sin(th1)*sin(th3)))/50, -(9*sin(th5)*(cos(th1)*cos(th4) + sin(th4)*(cos(th3)*cos(th2 + pi/2)*sin(th1) - sin(th1)*sin(th3)*sin(th2 + pi/2))))/50, - (9*cos(th5)*(cos(th1)*sin(th4) - cos(th4)*(cos(th3)*cos(th2 + pi/2)*sin(th1) - sin(th1)*sin(th3)*sin(th2 + pi/2))))/50 - (9*sin(th5)*(cos(th3)*sin(th1)*sin(th2 + pi/2) + cos(th2 + pi/2)*sin(th1)*sin(th3)))/50, 0]
% [                                                                                                                                                                                                                                                                                                                                                                                                                                          0,                                                                                  (17*cos(th2 + pi/2))/40 + (cos(th3)*cos(th2 + pi/2))/25 + (17*cos(th3)*sin(th2 + pi/2))/40 + (17*cos(th2 + pi/2)*sin(th3))/40 - (sin(th3)*sin(th2 + pi/2))/25 + (9*cos(th5)*(cos(th3)*sin(th2 + pi/2) + cos(th2 + pi/2)*sin(th3)))/50 + (9*cos(th4)*sin(th5)*(cos(th3)*cos(th2 + pi/2) - sin(th3)*sin(th2 + pi/2)))/50,                                                                         (cos(th3)*cos(th2 + pi/2))/25 + (17*cos(th3)*sin(th2 + pi/2))/40 + (17*cos(th2 + pi/2)*sin(th3))/40 - (sin(th3)*sin(th2 + pi/2))/25 + (9*cos(th5)*(cos(th3)*sin(th2 + pi/2) + cos(th2 + pi/2)*sin(th3)))/50 + (9*cos(th4)*sin(th5)*(cos(th3)*cos(th2 + pi/2) - sin(th3)*sin(th2 + pi/2)))/50,                                         -(9*sin(th4)*sin(th5)*(cos(th3)*sin(th2 + pi/2) + cos(th2 + pi/2)*sin(th3)))/50,                                                             (9*sin(th5)*(cos(th3)*cos(th2 + pi/2) - sin(th3)*sin(th2 + pi/2)))/50 + (9*cos(th4)*cos(th5)*(cos(th3)*sin(th2 + pi/2) + cos(th2 + pi/2)*sin(th3)))/50, 0]
% ];  










% viene chiamato J ma il jacobiano seguente è in verità il jacobiano di
% poszione Jp 
% J = [
% [(9*sin(th5)*(cos(th1)*sin(th4) - cos(th4)*(cos(th3)*cos(th2 + pi/2)*sin(th1) - sin(th1)*sin(th3)*sin(th2 + pi/2))))/100 - (17*cos(th2 + pi/2)*sin(th1))/40 - sin(th1)/20 - (9*cos(th5)*(cos(th3)*sin(th1)*sin(th2 + pi/2) + cos(th2 + pi/2)*sin(th1)*sin(th3)))/100 - (cos(th3)*cos(th2 + pi/2)*sin(th1))/25 - (17*cos(th3)*sin(th1)*sin(th2 + pi/2))/40 - (17*cos(th2 + pi/2)*sin(th1)*sin(th3))/40 + (sin(th1)*sin(th3)*sin(th2 + pi/2))/25, (17*cos(th1)*cos(th3)*cos(th2 + pi/2))/40 - (9*cos(th5)*(cos(th1)*sin(th3)*sin(th2 + pi/2) - cos(th1)*cos(th3)*cos(th2 + pi/2)))/100 - (cos(th1)*cos(th3)*sin(th2 + pi/2))/25 - (cos(th1)*cos(th2 + pi/2)*sin(th3))/25 - (17*cos(th1)*sin(th3)*sin(th2 + pi/2))/40 - (9*cos(th4)*sin(th5)*(cos(th1)*cos(th3)*sin(th2 + pi/2) + cos(th1)*cos(th2 + pi/2)*sin(th3)))/100 - (17*cos(th1)*sin(th2 + pi/2))/40, (17*cos(th1)*cos(th3)*cos(th2 + pi/2))/40 - (cos(th1)*cos(th3)*sin(th2 + pi/2))/25 - (cos(th1)*cos(th2 + pi/2)*sin(th3))/25 - (17*cos(th1)*sin(th3)*sin(th2 + pi/2))/40 - (9*cos(th4)*sin(th5)*(cos(th1)*cos(th3)*sin(th2 + pi/2) + cos(th1)*cos(th2 + pi/2)*sin(th3)))/100 - (9*cos(th5)*(cos(th1)*sin(th3)*sin(th2 + pi/2) - cos(th1)*cos(th3)*cos(th2 + pi/2)))/100,  (9*sin(th5)*(cos(th4)*sin(th1) + sin(th4)*(cos(th1)*sin(th3)*sin(th2 + pi/2) - cos(th1)*cos(th3)*cos(th2 + pi/2))))/100,   (9*cos(th5)*(sin(th1)*sin(th4) - cos(th4)*(cos(th1)*sin(th3)*sin(th2 + pi/2) - cos(th1)*cos(th3)*cos(th2 + pi/2))))/100 - (9*sin(th5)*(cos(th1)*cos(th3)*sin(th2 + pi/2) + cos(th1)*cos(th2 + pi/2)*sin(th3)))/100, 0]
% [cos(th1)/20 + (17*cos(th1)*cos(th2 + pi/2))/40 + (9*sin(th5)*(sin(th1)*sin(th4) - cos(th4)*(cos(th1)*sin(th3)*sin(th2 + pi/2) - cos(th1)*cos(th3)*cos(th2 + pi/2))))/100 + (9*cos(th5)*(cos(th1)*cos(th3)*sin(th2 + pi/2) + cos(th1)*cos(th2 + pi/2)*sin(th3)))/100 + (17*cos(th1)*cos(th3)*sin(th2 + pi/2))/40 + (17*cos(th1)*cos(th2 + pi/2)*sin(th3))/40 - (cos(th1)*sin(th3)*sin(th2 + pi/2))/25 + (cos(th1)*cos(th3)*cos(th2 + pi/2))/25, (9*cos(th5)*(cos(th3)*cos(th2 + pi/2)*sin(th1) - sin(th1)*sin(th3)*sin(th2 + pi/2)))/100 - (17*sin(th1)*sin(th2 + pi/2))/40 + (17*cos(th3)*cos(th2 + pi/2)*sin(th1))/40 - (cos(th3)*sin(th1)*sin(th2 + pi/2))/25 - (cos(th2 + pi/2)*sin(th1)*sin(th3))/25 - (17*sin(th1)*sin(th3)*sin(th2 + pi/2))/40 - (9*cos(th4)*sin(th5)*(cos(th3)*sin(th1)*sin(th2 + pi/2) + cos(th2 + pi/2)*sin(th1)*sin(th3)))/100, (9*cos(th5)*(cos(th3)*cos(th2 + pi/2)*sin(th1) - sin(th1)*sin(th3)*sin(th2 + pi/2)))/100 + (17*cos(th3)*cos(th2 + pi/2)*sin(th1))/40 - (cos(th3)*sin(th1)*sin(th2 + pi/2))/25 - (cos(th2 + pi/2)*sin(th1)*sin(th3))/25 - (17*sin(th1)*sin(th3)*sin(th2 + pi/2))/40 - (9*cos(th4)*sin(th5)*(cos(th3)*sin(th1)*sin(th2 + pi/2) + cos(th2 + pi/2)*sin(th1)*sin(th3)))/100, -(9*sin(th5)*(cos(th1)*cos(th4) + sin(th4)*(cos(th3)*cos(th2 + pi/2)*sin(th1) - sin(th1)*sin(th3)*sin(th2 + pi/2))))/100, - (9*cos(th5)*(cos(th1)*sin(th4) - cos(th4)*(cos(th3)*cos(th2 + pi/2)*sin(th1) - sin(th1)*sin(th3)*sin(th2 + pi/2))))/100 - (9*sin(th5)*(cos(th3)*sin(th1)*sin(th2 + pi/2) + cos(th2 + pi/2)*sin(th1)*sin(th3)))/100, 0]
% [                                                                                                                                                                                                                                                                                                                                                                                                                                            0,                                                                                  (17*cos(th2 + pi/2))/40 + (cos(th3)*cos(th2 + pi/2))/25 + (17*cos(th3)*sin(th2 + pi/2))/40 + (17*cos(th2 + pi/2)*sin(th3))/40 - (sin(th3)*sin(th2 + pi/2))/25 + (9*cos(th5)*(cos(th3)*sin(th2 + pi/2) + cos(th2 + pi/2)*sin(th3)))/100 + (9*cos(th4)*sin(th5)*(cos(th3)*cos(th2 + pi/2) - sin(th3)*sin(th2 + pi/2)))/100,                                                                         (cos(th3)*cos(th2 + pi/2))/25 + (17*cos(th3)*sin(th2 + pi/2))/40 + (17*cos(th2 + pi/2)*sin(th3))/40 - (sin(th3)*sin(th2 + pi/2))/25 + (9*cos(th5)*(cos(th3)*sin(th2 + pi/2) + cos(th2 + pi/2)*sin(th3)))/100 + (9*cos(th4)*sin(th5)*(cos(th3)*cos(th2 + pi/2) - sin(th3)*sin(th2 + pi/2)))/100,                                         -(9*sin(th4)*sin(th5)*(cos(th3)*sin(th2 + pi/2) + cos(th2 + pi/2)*sin(th3)))/100,                                                             (9*sin(th5)*(cos(th3)*cos(th2 + pi/2) - sin(th3)*sin(th2 + pi/2)))/100 + (9*cos(th4)*cos(th5)*(cos(th3)*sin(th2 + pi/2) + cos(th2 + pi/2)*sin(th3)))/100, 0]
% ];

== matlab function Modello_Irb1300/MATLAB Function2 ==
  data: t input; P output; O_d output; mode input
function [P,O_d] = trapezioPlanner(t,mode)
    % Parametri per la traiettoria
    % Tempo di pianificazione
    % ogni tappa è definita come: 
    % struct('Pi', [Posizione inizale end effector], 'Pf', [posizione
    % finale end effector], 'tf', [durata della tappa], 'tw',[tempo di attesa a fine tappa],'O',[orientazione end effector]),
    %
    %struct('Pi', [X ; Y; Z], 'Pf', [X ; Y; Z], 'tf', [secondi], 'tw',[secondi],'O',[asse di rotazione X, asse di rotazione Y, asse di rotazione Z]),
    steps = [
            struct('Pi', [0.66; 1.015;   0], 'Pf', [0.55; 0.72; 0.45], 'tf', 15, 'tw', 5,'O',  [0, 0, 0]),        % Tappa 1
            struct('Pi', [0.55; 0.73; 0.45], 'Pf', [0.60; 0.70; 0.40], 'tf',  6, 'tw', 2,'O',  [0, 0, 0]),        % Tappa 2
            struct('Pi', [0.60; 0.70; 0.40], 'Pf', [0.55; 0.70; 0.40], 'tf',  6, 'tw', 2,'O',  [0, 0,-pi/2]),     % Tappa 3
            struct('Pi', [0.55; 0.70; 0.40], 'Pf', [0.55; 0.57; 0.14], 'tf', 15, 'tw', 5,'O',  [0, 0,-pi/2]),     % Tappa 4 
            struct('Pi', [0.55; 0.57; 0.14], 'Pf', [0.45; 0.57; 0.14], 'tf', 16, 'tw', 5,'O',  [0, 0,-pi/2])      % Tappa 4
            ];
    switch mode
        case 0
            steps = [
            struct('Pi', [0.66; 1.010;   0], 'Pf', [0.55; 0.72; 0.45], 'tf', 4, 'tw', 0.01,'O',  [0, 0, 0]),        % Tappa 1
            struct('Pi', [0.55; 0.73; 0.45], 'Pf', [0.60; 0.70; 0.40], 'tf', 4, 'tw', 0.01,'O',  [0, 0, 0]),        % Tappa 2
            struct('Pi', [0.60; 0.70; 0.40], 'Pf', [0.55; 0.70; 0.40], 'tf', 4, 'tw', 0.01,'O',  [0, 0,-pi/2]),     % Tappa 3
            struct('Pi', [0.55; 0.70; 0.40], 'Pf', [0.55; 0.57; 0.14], 'tf', 4, 'tw', 0.01,'O',  [0, 0,-pi/2]),     % Tappa 4 
            struct('Pi', [0.55; 0.57; 0.14], 'Pf', [0.45; 0.57; 0.14], 'tf', 4, 'tw', 0.01,'O',  [0, 0,-pi/2]),     % Tappa 5
            struct('Pi', [0.45; 0.57; 0.14], 'Pf', [0.66; 1.010;   0], 'tf', 16, 'tw', 0.95,'O',  [0, 0, 0])         % Tappa 6
            ];

        case 1
            steps = [
            struct('Pi', [0.66; 1.010;   0], 'Pf', [0.45; 0.57; 0.14], 'tf', 4, 'tw', 0.01,'O',  [0, 0, 0]),        % Tappa 1
            struct('Pi', [0.45; 0.57; 0.14], 'Pf', [0.55; 0.57; 0.14], 'tf', 4, 'tw', 0.01,'O',  [0, 0, -pi/2]),    % Tappa 2
            struct('Pi', [0.55; 0.57; 0.14], 'Pf', [0.55; 0.57; 0.20], 'tf', 4, 'tw', 0.01,'O',  [0, 0, -pi/2]),    % Tappa 3
            struct('Pi', [0.55; 0.57; 0.20], 'Pf', [0.55; 0.80; 0.40], 'tf', 4, 'tw', 0.01,'O',  [0, 0, -pi/2]),    % Tappa 4 
            struct('Pi', [0.55; 0.80; 0.40], 'Pf', [0.55; 0.70; 0.45], 'tf', 4, 'tw', 0.01,'O',  [0, 0, 0]),        % Tappa 5
            struct('Pi', [0.55; 0.70; 0.45], 'Pf', [0.50; 0.70; 0.45], 'tf', 4, 'tw', 0.01,'O',  [0, 0, 0]),        % Tappa 6
            struct('Pi', [0.50; 0.70; 0.45], 'Pf', [0.66; 1.010; 0], 'tf',   6, 'tw', 6.9,'O',  [0, 0, 0])         % Tappa 7
            ];
    end
    
   
    % Inizializzazione del tempo accumulato
    t_accum = 0; 
    
    % Matrice di trasformazione scena -> robot
    R_scene_to_robot = [ 1, 0,  0;   % x_s -> x_r
                         0, 0, -1;   % z_s -> -y_r
                         0, 1,  0];  % y_s -> z_r

    % Inizializzazione della posizione nello spazio scena
    
    P_scene = steps(1).Pi; % Posizione iniziale come fallback
    O_d = steps(1).O;      % orientazione iniziale come fallback
   
  % Calcolo della traiettoria lineare per ciascuna tappa
    for i = 1:length(steps)
        step = steps(i);
        
        % impostazione dell'orientazione dsiderata 
        O_d = step.O;

        % Tempo di inizio e fine della tappa
        t_start = t_accum;
        t_end = t_start + step.tf;
        
        % Controlla se il tempo attuale appartiene alla tappa corrente
        if t >= t_start && t < t_end
            % Calcola accelerazione
            delta_P = step.Pf - step.Pi;
            Acc = 4 * delta_P / step.tf^2; % Accelerazione necessaria

            % Calcola i tempi critici per il profilo trapezoidale
            sqrtTerm = sqrt(step.tf^2 / 4 - norm(delta_P) / norm(Acc));
            tc1 = step.tf / 2 - sqrtTerm;
            tc2 = step.tf / 2 + sqrtTerm;
            
            t_rel = t - t_start;

            % Calcolo posizione in base al profilo trapezoidale
            if t_rel >= 0 && t_rel < tc1
                % Fase di accelerazione
                P_scene = step.Pi + 1/2 * Acc * t_rel^2;
                
            elseif t_rel >= tc1 && t_rel < tc2
                % Fase a velocità costante
                P_scene = step.Pi + Acc * tc1 * (t_rel - tc1 / 2);
                
            elseif t_rel >= tc2 && t_rel < step.tf
                % Fase di decelerazione
                P_scene = step.Pf - 1/2 * Acc * (step.tf - t_rel)^2;
                
            end

            break; % Interrompe il loop dopo aver trovato la tappa corrente
        elseif t >= t_end && t < t_end + step.tw
            % Fase di attesa (mantiene la posizione finale della tappa)
            P_scene = step.Pf;
            break; % Interrompe il loop
        end

        % Aggiorna il tempo accumulato per la prossima tappa
        t_accum = t_end + step.tw;
    end
    
    % Conversione in coordinate robot
    position_robot = R_scene_to_robot * P_scene;
    % Uscita: combinazione di posizione, orientamento, velocità e accelerazioni
    P = [position_robot];
    %O_d = [theta,phi,psi];  % Rotazione attorno all'asse x 
    % Rotazione attorno all'asse y 
           
end
% % Funzione per calcolare i tempi critici
% function [tc1, tc2] = calculateCriticalTimes(delta_P, Acc, tf)
%     % Calcolo dei tempi critici per traiettoria a trapezio
%     sqrtTerm = sqrt(tf^2 / 4 - norm(delta_P) / norm(Acc));
%     tc1 = tf / 2 - sqrtTerm;
%     tc2 = tf / 2 + sqrtTerm;
% end






% function P = trapezioPlanner(t)
%     % Parametri per la traiettoria
%     % Tempo di pianificazione
% 
%     ti = 0;
%     tf1 = 10; % Tempo finale della prima tappa
%     tw = 10;   % Tempo di attesa tra le tappe
%     tf2_start = tf1 + tw; % Inizio seconda traiettoria
%     tf2 = 40 + tw; % Fine seconda tappa (durata estesa)
% 
%     % Definizione delle posizioni iniziali e finali nello spazio scena
%     Pi1_scene = [0.60; 0.7; 0.4];      % Posizione iniziale prima tappa (scena)
%     Pf1_scene = [0.60; 0.7; 0.4];     % Posizione finale prima tappa (scena)
%     Pi2_scene = Pf1_scene;             % Posizione iniziale seconda tappa (scena)
%     Pf2_scene = [0.40; 0.8; 0];      % Posizione finale seconda tappa (scena)
%     P_scene = Pi1_scene;
% 
%     % % Orientamento nello spazio scena (variazione per test)
%     % RPY_start = [1.57;0;0]; % Orientamento iniziale in RPY
%     % RPY_end = [1.57;0;0];    % Orientamento finale in RPY
%     % RPY_scene = RPY_start;
% 
%     % Matrice di trasformazione scena -> robot per le posizioni
%     R_scene_to_robot = [ 1, 0,  0;   % x_s -> x_r
%                          0, 0, -1;   % z_s -> -y_r
%                          0, 1,  0];  % y_s -> z_r
% 
%     % Tempo relativo per la traiettoria
%     t_rel = t;
% 
%     % Calcolo della traiettoria lineare
%     if t_rel >= 0 && t_rel < tf1
%         % Prima tappa
%         Acc1 = (4 * (Pf1_scene - Pi1_scene) / (tf1^2)) * 1.1; % Accelerazione
%         delta_P1 = Pf1_scene - Pi1_scene;
%         tc1_1 = tf1 / 2 - sqrt(tf1^2 / 4 - norm(delta_P1) / norm(Acc1));
%         tc2_1 = tf1 / 2 + sqrt(tf1^2 / 4 - norm(delta_P1) / norm(Acc1));
% 
%         if t_rel >= 0 && t_rel < tc1_1
%             % Accelerazione lineare
%             P_scene = Pi1_scene + 1/2 * Acc1 * t_rel^2;
% 
%         elseif t_rel >= tc1_1 && t_rel < tc2_1
%             % Velocità costante
%             P_scene = Pi1_scene + Acc1 * tc1_1 * (t_rel - tc1_1 / 2);
% 
%         elseif t_rel >= tc2_1 && t_rel < tf1
%             % Decelerazione lineare
%             P_scene = Pf1_scene - 1/2 * Acc1 * (tf1 - t_rel)^2;
% 
%         end
%     elseif t_rel >= tf1 && t_rel < tf2_start
%         % Tempo di attesa
%         P_scene = Pf1_scene; % Mantiene la posizione finale della prima tappa
% 
%     elseif t_rel >= tf2_start && t_rel < tf2
%         % Seconda tappa
%         Acc2 = (4 * (Pf2_scene - Pi2_scene) / ((tf2 - tf2_start)^2)) * 1.1; % Accelerazione
%         delta_P2 = Pf2_scene - Pi2_scene;
%         t2_duration = tf2 - tf2_start;
%         tc1_2 = t2_duration / 2 - sqrt(t2_duration^2 / 4 - norm(delta_P2) / norm(Acc2));
%         tc2_2 = t2_duration / 2 + sqrt(t2_duration^2 / 4 - norm(delta_P2) / norm(Acc2));
%         t_rel2 = t_rel - tf2_start; % Tempo relativo alla seconda tappa
% 
%         if t_rel2 >= 0 && t_rel2 < tc1_2
%             % Accelerazione lineare
%             P_scene = Pi2_scene + 1/2 * Acc2 * t_rel2^2;
% 
%         elseif t_rel2 >= tc1_2 && t_rel2 < tc2_2
%             % Velocità costante
%             P_scene = Pi2_scene + Acc2 * tc1_2 * (t_rel2 - tc1_2 / 2);
% 
%         elseif t_rel2 >= tc2_2 && t_rel2 < t2_duration
%             % Decelerazione lineare
%             P_scene = Pf2_scene - 1/2 * Acc2 * (t2_duration - t_rel2)^2;
% 
%         end
%     else
%         % Fine della traiettoria
%         P_scene = Pf2_scene;
% 
%     end
% 
% 
%     position_robot = R_scene_to_robot * P_scene;
%     % Uscita: combinazione di posizione, orientamento, velocità e accelerazioni
%     %P = [position_robot; orientation_robot];
%     P = [position_robot];
% end
